simulink model "StepA_model"  (R2025b)
settings: Solver=FixedStepAuto  StartTime=0.0  StopTime=10.0  RelTol=1e-3
undefined symbols (not defined in the file or in its folder): netA_export
libraries: dlconvfclib x4, dlsequencelib x1, dlactivationlib x1
settings Model: Creator=10932  LastModifiedBy=10932
settings OptimizationCC: DefaultParameterBehavior=Inlined  EnhancedBackFolding=on  PassReuseOutputArgsAs=Individual arguments  ZeroExternalMemoryAtStartup=off  ZeroInternalMemoryAtStartup=off  OptimizeBlockOrder=speed  DifferentSizesBufferReuse=on  OptimizationCustomize=off  EfficientTunableParamExpr=on
settings DebuggingCC: ParameterTunabilityLossMsg=error
settings SFSimCC: MATLABDynamicMemAlloc=off
settings RTWCC: SystemTargetFile=ert.tlc  TemplateMakefile=ert_default_tmf  Description=Embedded Coder
settings CodeAppCC: ForceParamTrailComments=on  IgnoreCustomStorageClasses=off  OperatorAnnotations=on  SimulinkDataObjDesc=on  SFDataObjDesc=on  InsertBlockDesc=on
settings ERTTargetCC: ERTCustomFileTemplate=example_file_process.tlc  TargetLangStandard=C99 (ISO)  GenerateSampleERTMain=on

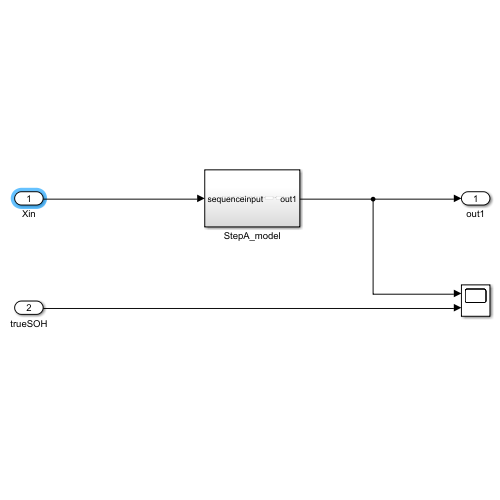
[thumbnail: Simulink's stored preview of the top-level diagram]
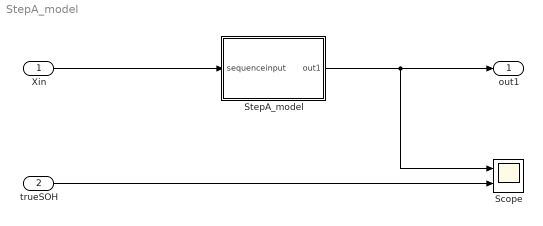
== system StepA_model ==
  Xin : Inport  PortDimensions="[4  1]"  Interpolate=off
  trueSOH : Inport  Port=2
  Scope : Scope  NumInputPorts=2
  StepA_model : Subsystem
  out1 : Outport
  wires:
  Xin/1 -> StepA_model/1(sequenceinput)
  trueSOH/1 -> Scope/2
  StepA_model/1(out1) -> Scope/1, out1/1

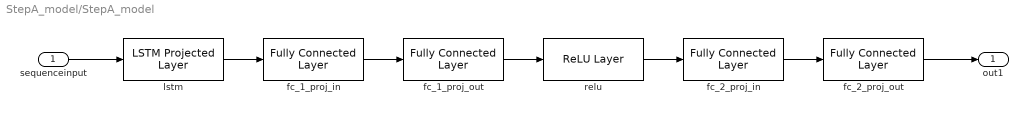
== system StepA_model/StepA_model ==
  sequenceinput : Inport  PortDimensions="[4  1]"
  fc_1_proj_in : dlconvfclib/Fully Connected Layer  Layer=netA_export.Layers(3)  OutMin=[]  OutMax=[]  WeightsDataTypeStr=Inherit: Inherit via back propagation  WeightsMin=[]  WeightsMax=[]  BiasDataTypeStr=Inherit: Inherit via back propagation  BiasMin=[]  BiasMax=[]  AccumMin=[]  AccumMax=[]  InternalRndMeth=Floor  InternalSaturateOnIntegerOverflow=off  SampleTime=-1
      settings: DataFormat=C
  fc_1_proj_out : dlconvfclib/Fully Connected Layer  Layer=netA_export.Layers(4)  OutMin=[]  OutMax=[]  WeightsDataTypeStr=Inherit: Inherit via back propagation  WeightsMin=[]  WeightsMax=[]  BiasDataTypeStr=Inherit: Inherit via back propagation  BiasMin=[]  BiasMax=[]  AccumMin=[]  AccumMax=[]  InternalRndMeth=Floor  InternalSaturateOnIntegerOverflow=off  SampleTime=-1
      settings: DataFormat=C
  fc_2_proj_in : dlconvfclib/Fully Connected Layer  Layer=netA_export.Layers(6)  OutMin=[]  OutMax=[]  WeightsDataTypeStr=Inherit: Inherit via back propagation  WeightsMin=[]  WeightsMax=[]  BiasDataTypeStr=Inherit: Inherit via back propagation  BiasMin=[]  BiasMax=[]  AccumMin=[]  AccumMax=[]  InternalRndMeth=Floor  InternalSaturateOnIntegerOverflow=off  SampleTime=-1
      settings: DataFormat=C
  fc_2_proj_out : dlconvfclib/Fully Connected Layer  Layer=netA_export.Layers(7)  OutMin=[]  OutMax=[]  WeightsDataTypeStr=Inherit: Inherit via back propagation  WeightsMin=[]  WeightsMax=[]  BiasDataTypeStr=Inherit: Inherit via back propagation  BiasMin=[]  BiasMax=[]  AccumMin=[]  AccumMax=[]  InternalRndMeth=Floor  InternalSaturateOnIntegerOverflow=off  SampleTime=-1
      settings: DataFormat=C
  lstm : dlsequencelib/LSTM Projected Layer  Layer=netA_export.Layers(2)  Stateful=off  ApproximationMethod=None  OutMin=[]  OutMax=[]  InputWeightsDataTypeStr=Inherit: Inherit via back propagation  InputWeightsMin=[]  InputWeightsMax=[]  RecurrentWeightsDataTypeStr=Inherit: Inherit via back propagation  RecurrentWeightsMin=[]  RecurrentWeightsMax=[]  BiasDataTypeStr=Inherit: Inherit via back propagation  BiasMin=[]  BiasMax=[]  InputProjectorWeightsDataTypeStr=Inherit: Inherit via back propagation  InputProjectorWeightsMin=[]  InputProjectorWeightsMax=[]  OutputProjectorWeightsDataTypeStr=Inherit: Inherit via back propagation  OutputProjectorWeightsMin=[]  OutputProjectorWeightsMax=[]  InitialCellStateDataTypeStr=Inherit: Inherit via back propagation  InitialCellStateMin=[]  InitialCellStateMax=[]  CellStateMin=[]  CellStateMax=[]  InitialHiddenStateDataTypeStr=Inherit: Inherit via back propagation  InitialHiddenStateMin=[]  InitialHiddenStateMax=[]  HiddenStateMin=[]  HiddenStateMax=[]  InputWeightsMatrixMultiplyOutMin=[]  InputWeightsMatrixMultiplyOutMax=[]  RecurrentWeightsMatrixMultiplyOutMin=[]  RecurrentWeightsMatrixMultiplyOutMax=[]  InputProjectorWeightsMatrixMultiplyOutMin=[]  InputProjectorWeightsMatrixMultiplyOutMax=[]  OutputProjectorWeightsMatrixMultiplyOutMin=[]  OutputProjectorWeightsMatrixMultiplyOutMax=[]  LinearGateAddOutMin=[]  LinearGateAddOutMax=[]  CellStateProductOutMin=[]  CellStateProductOutMax=[]  SampleTime=-1
      settings: DataFormat=CT
  relu : dlactivationlib/ReLU Layer  OutMin=[]  OutMax=[]  SampleTime=-1
  out1 : Outport
  wires:
  fc_1_proj_in/1 -> fc_1_proj_out/1
  sequenceinput/1 -> lstm/1
  fc_1_proj_out/1 -> relu/1
  fc_2_proj_in/1 -> fc_2_proj_out/1
  lstm/1 -> fc_1_proj_in/1
  relu/1 -> fc_2_proj_in/1
  fc_2_proj_out/1 -> out1/1
